simulink subsystem "RX"  (R2022b)
settings: Solver=VariableStepAuto  StartTime=0.0  StopTime=10.0  RelTol=1e-3
libraries: msbPllFoundation x2
settings Model: Creator=Ali-Laptop  LastModifiedBy=Ali-Laptop

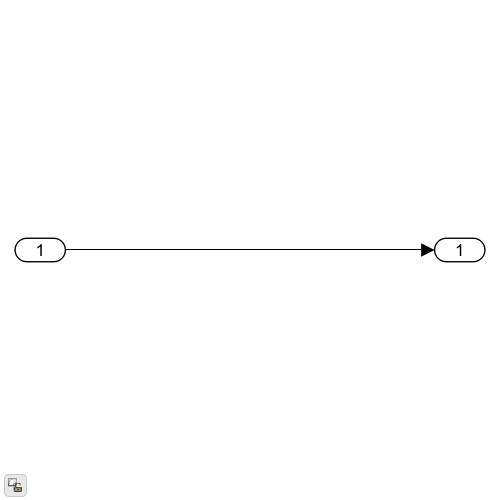
[thumbnail: Simulink's stored preview of the top-level diagram]
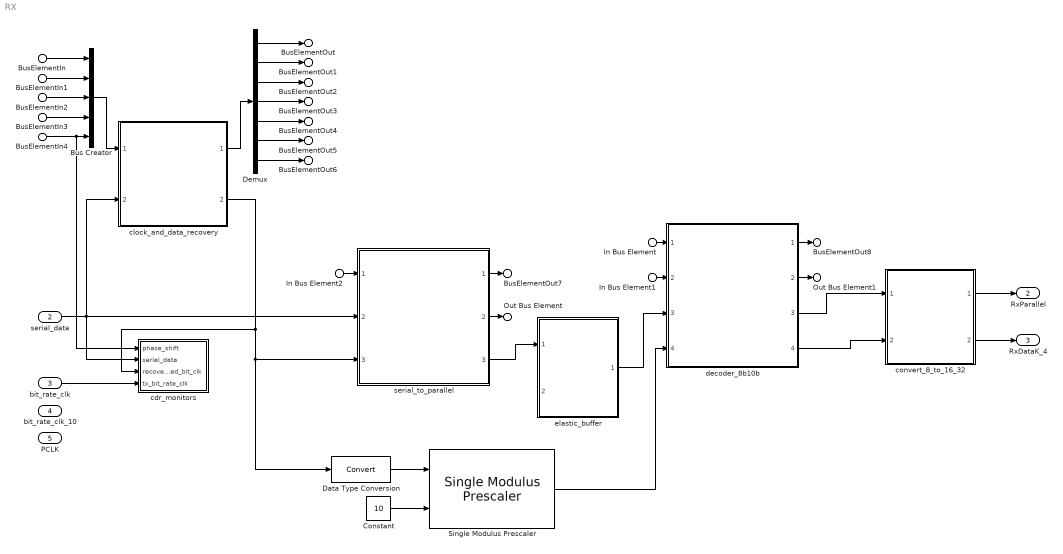
== system RX ==
  In Bus Element : Inport  PortName=digital_out  Element=RxDataK_out
  In Bus Element1 : Inport  PortName=digital_out  Element=RxParallel_8_out
  In Bus Element2 : Inport  PortName=digital_out  Element=RxParallel_10_out
  BusElementIn : Inport  PortName=digital_out  Element=Dn_out
  BusElementIn1 : Inport  PortName=digital_out  Element=Dn_1_out
  BusElementIn2 : Inport  PortName=digital_out  Element=Pn_out
  BusElementIn3 : Inport  PortName=digital_out  Element=decision_out
  BusElementIn4 : Inport  PortName=digital_out  Element=phase_shift
  serial_data : Inport  Port=2
  bit_rate_clk : Inport  Port=3
  bit_rate_clk_10 : Inport  Port=4
  PCLK : Inport  Port=5
  Bus Creator : BusCreator  Inputs=5
  Constant : Constant  Value=10
  Data Type Conversion : DataTypeConversion  SaturateOnIntegerOverflow=off  RndMeth=Floor
  Demux : Demux  Outputs=7
  Single Modulus Prescaler : msbPllFoundation/Single Modulus Prescaler  ExtraBuffer=off  NBuffer=1
  cdr_monitors : Subsystem
  clock_and_data_recovery : Subsystem  ReferencedSubsystem=clock_and_data_recovery
  convert_8_to_16_32 : Subsystem  ReferencedSubsystem=convert_8_to_16_32
  decoder_8b10b : Subsystem  ReferencedSubsystem=decoder_8b10b
  elastic_buffer : Subsystem  ReferencedSubsystem=elastic_buffer
  serial_to_parallel : Subsystem  ReferencedSubsystem=serial_to_parallel
  BusElementOut7 : Outport  PortName=digital_in  Element=RxBitCLK
  BusElementOut8 : Outport  PortName=digital_in  Element=RxBitCLK_10
  Out Bus Element : Outport  PortName=digital_in  Element=Serial_in
  Out Bus Element1 : Outport  PortName=digital_in  Element=RxParallel_10_in
  BusElementOut : Outport  PortName=digital_in  Element=data_clock
  BusElementOut1 : Outport  PortName=digital_in  Element=phase_clock
  BusElementOut2 : Outport  PortName=digital_in  Element=Dn_in
  BusElementOut3 : Outport  PortName=digital_in  Element=Dn_1_in
  BusElementOut4 : Outport  PortName=digital_in  Element=Pn_in
  BusElementOut5 : Outport  PortName=digital_in  Element=decision_in
  BusElementOut6 : Outport  PortName=digital_in  Element=recovered_clock
  RxParallel : Outport  Port=2
  RxDataK_4 : Outport  Port=3
  wires:
  elastic_buffer/1 -> decoder_8b10b/3
  convert_8_to_16_32/1 -> RxParallel/1
  clock_and_data_recovery/2 -> cdr_monitors/3(recovered_bit_clk), serial_to_parallel/3, Data Type Conversion/1
  serial_data/1 -> serial_to_parallel/2, cdr_monitors/2(serial_data), clock_and_data_recovery/2
  serial_to_parallel/2 -> Out Bus Element/1
  In Bus Element2/1 -> serial_to_parallel/1
  decoder_8b10b/2 -> Out Bus Element1/1
  decoder_8b10b/3 -> convert_8_to_16_32/1
  decoder_8b10b/4 -> convert_8_to_16_32/2
  In Bus Element/1 -> decoder_8b10b/1
  In Bus Element1/1 -> decoder_8b10b/2
  convert_8_to_16_32/2 -> RxDataK_4/1
  serial_to_parallel/3 -> elastic_buffer/1
  BusElementIn/1 -> Bus Creator/1
  BusElementIn1/1 -> Bus Creator/2
  BusElementIn2/1 -> Bus Creator/3
  BusElementIn3/1 -> Bus Creator/4
  BusElementIn4/1 -> Bus Creator/5, cdr_monitors/1(phase_shift)
  Bus Creator/1 -> clock_and_data_recovery/1
  Demux/1 -> BusElementOut/1
  Demux/2 -> BusElementOut1/1
  Demux/3 -> BusElementOut2/1
  Demux/4 -> BusElementOut3/1
  Demux/5 -> BusElementOut4/1
  Demux/6 -> BusElementOut5/1
  serial_to_parallel/1 -> BusElementOut7/1
  clock_and_data_recovery/1 -> Demux/1
  Demux/7 -> BusElementOut6/1
  decoder_8b10b/1 -> BusElementOut8/1
  Single Modulus Prescaler/1 -> decoder_8b10b/4
  Constant/1 -> Single Modulus Prescaler/2
  Data Type Conversion/1 -> Single Modulus Prescaler/1
  bit_rate_clk/1 -> cdr_monitors/4(tx_bit_rate_clk)

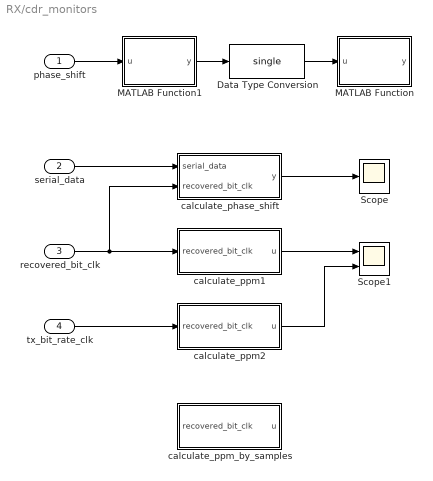
== system RX/cdr_monitors ==
  phase_shift : Inport
  serial_data : Inport  Port=2
  recovered_bit_clk : Inport  Port=3
  tx_bit_rate_clk : Inport  Port=4
  Data Type Conversion : DataTypeConversion  OutDataTypeStr=single  SaturateOnIntegerOverflow=off  RndMeth=Floor
  MATLAB Function : MATLAB Function  TreatAsAtomicUnit=on
  MATLAB Function1 : MATLAB Function  TreatAsAtomicUnit=on
  Scope : Scope
  Scope1 : Scope  NumInputPorts=2
  calculate_phase_shift : Subsystem
  calculate_ppm1 : Subsystem
  calculate_ppm2 : Subsystem
  calculate_ppm_by_samples : Subsystem
  wires:
  calculate_ppm2/1(u) -> Scope1/2
  tx_bit_rate_clk/1 -> calculate_ppm2/1(recovered_bit_clk)
  calculate_ppm1/1(u) -> Scope1/1
  Data Type Conversion/1 -> MATLAB Function/1(u)
  phase_shift/1 -> MATLAB Function1/1(u)
  MATLAB Function1/1(y) -> Data Type Conversion/1
  calculate_phase_shift/1(y) -> Scope/1
  recovered_bit_clk/1 -> calculate_ppm1/1(recovered_bit_clk), calculate_phase_shift/2(recovered_bit_clk)
  serial_data/1 -> calculate_phase_shift/1(serial_data)

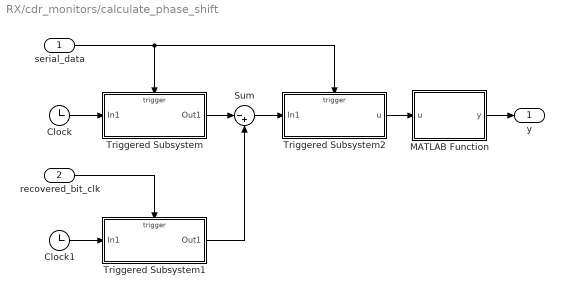
== system RX/cdr_monitors/calculate_phase_shift ==
  serial_data : Inport
  recovered_bit_clk : Inport  Port=2
  Clock : Clock
  Clock1 : Clock
  MATLAB Function : MATLAB Function  TreatAsAtomicUnit=on
  Sum : Sum  Inputs=|-+
  Triggered Subsystem : Subsystem  TreatAsAtomicUnit=on
  Triggered Subsystem1 : Subsystem  TreatAsAtomicUnit=on
  Triggered Subsystem2 : Subsystem  TreatAsAtomicUnit=on
  y : Outport
  wires:
  Triggered Subsystem2/1(u) -> MATLAB Function/1(u)
  MATLAB Function/1(y) -> y/1
  Sum/1 -> Triggered Subsystem2/1(In1)
  Triggered Subsystem1/1(Out1) -> Sum/2
  Triggered Subsystem/1(Out1) -> Sum/1
  serial_data/1 -> Triggered Subsystem/Trigger, Triggered Subsystem2/Trigger
  recovered_bit_clk/1 -> Triggered Subsystem1/Trigger
  Clock1/1 -> Triggered Subsystem1/1(In1)
  Clock/1 -> Triggered Subsystem/1(In1)

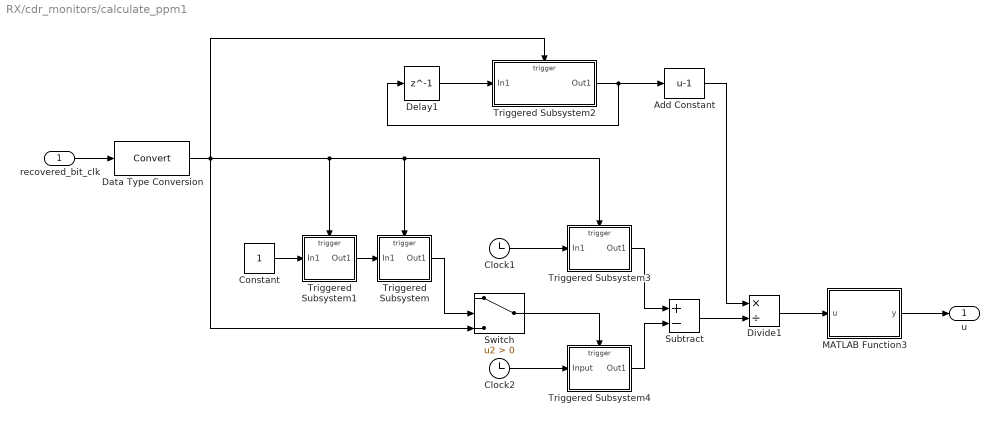
== system RX/cdr_monitors/calculate_ppm1 ==
  recovered_bit_clk : Inport
  Add Constant : Bias  Bias=-1  SaturateOnIntegerOverflow=off
  Clock1 : Clock
  Clock2 : Clock
  Constant : Constant
  Data Type Conversion : DataTypeConversion  SaturateOnIntegerOverflow=off  RndMeth=Floor
  Delay1 : Delay  DelayLength=1
  Divide1 : Product  Inputs=*/
  MATLAB Function3 : MATLAB Function  TreatAsAtomicUnit=on
  Subtract : Sum  Inputs=+-
  Switch : Switch  Criteria=u2 > Threshold  SaturateOnIntegerOverflow=off  InputSameDT=off
  Triggered Subsystem : Subsystem  TreatAsAtomicUnit=on
  Triggered Subsystem1 : Subsystem  TreatAsAtomicUnit=on
  Triggered Subsystem2 : Subsystem  TreatAsAtomicUnit=on
  Triggered Subsystem3 : Subsystem  TreatAsAtomicUnit=on
  Triggered Subsystem4 : Subsystem  TreatAsAtomicUnit=on
  u : Outport
  wires:
  Constant/1 -> Triggered Subsystem1/1(In1)
  MATLAB Function3/1(y) -> u/1
  Triggered Subsystem/1(Out1) -> Switch/2
  Triggered Subsystem1/1(Out1) -> Triggered Subsystem/1(In1)
  Divide1/1 -> MATLAB Function3/1(u)
  Data Type Conversion/1 -> Triggered Subsystem2/Trigger, Triggered Subsystem/Trigger, Triggered Subsystem3/Trigger, Triggered Subsystem1/Trigger, Switch/3
  Delay1/1 -> Triggered Subsystem2/1(In1)
  Triggered Subsystem4/1(Out1) -> Subtract/2
  Clock2/1 -> Triggered Subsystem4/1(Input)
  Switch/1 -> Triggered Subsystem4/Trigger
  Add Constant/1 -> Divide1/1
  recovered_bit_clk/1 -> Data Type Conversion/1
  Clock1/1 -> Triggered Subsystem3/1(In1)
  Triggered Subsystem3/1(Out1) -> Subtract/1
  Triggered Subsystem2/1(Out1) -> Add Constant/1, Delay1/1
  Subtract/1 -> Divide1/2

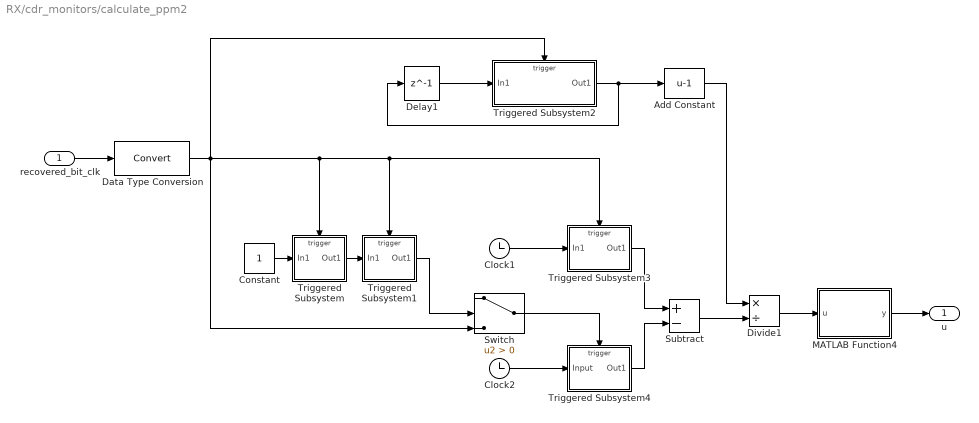
== system RX/cdr_monitors/calculate_ppm2 ==
  recovered_bit_clk : Inport
  Add Constant : Bias  Bias=-1  SaturateOnIntegerOverflow=off
  Clock1 : Clock
  Clock2 : Clock
  Constant : Constant
  Data Type Conversion : DataTypeConversion  SaturateOnIntegerOverflow=off  RndMeth=Floor
  Delay1 : Delay  DelayLength=1
  Divide1 : Product  Inputs=*/
  MATLAB Function4 : MATLAB Function  TreatAsAtomicUnit=on
  Subtract : Sum  Inputs=+-
  Switch : Switch  Criteria=u2 > Threshold  SaturateOnIntegerOverflow=off  InputSameDT=off
  Triggered Subsystem : Subsystem  TreatAsAtomicUnit=on
  Triggered Subsystem1 : Subsystem  TreatAsAtomicUnit=on
  Triggered Subsystem2 : Subsystem  TreatAsAtomicUnit=on
  Triggered Subsystem3 : Subsystem  TreatAsAtomicUnit=on
  Triggered Subsystem4 : Subsystem  TreatAsAtomicUnit=on
  u : Outport
  wires:
  MATLAB Function4/1(y) -> u/1
  Triggered Subsystem/1(Out1) -> Triggered Subsystem1/1(In1)
  Triggered Subsystem1/1(Out1) -> Switch/2
  Constant/1 -> Triggered Subsystem/1(In1)
  Divide1/1 -> MATLAB Function4/1(u)
  Data Type Conversion/1 -> Triggered Subsystem2/Trigger, Triggered Subsystem/Trigger, Triggered Subsystem3/Trigger, Triggered Subsystem1/Trigger, Switch/3
  Delay1/1 -> Triggered Subsystem2/1(In1)
  Triggered Subsystem4/1(Out1) -> Subtract/2
  Clock2/1 -> Triggered Subsystem4/1(Input)
  Switch/1 -> Triggered Subsystem4/Trigger
  Add Constant/1 -> Divide1/1
  recovered_bit_clk/1 -> Data Type Conversion/1
  Clock1/1 -> Triggered Subsystem3/1(In1)
  Triggered Subsystem3/1(Out1) -> Subtract/1
  Triggered Subsystem2/1(Out1) -> Add Constant/1, Delay1/1
  Subtract/1 -> Divide1/2

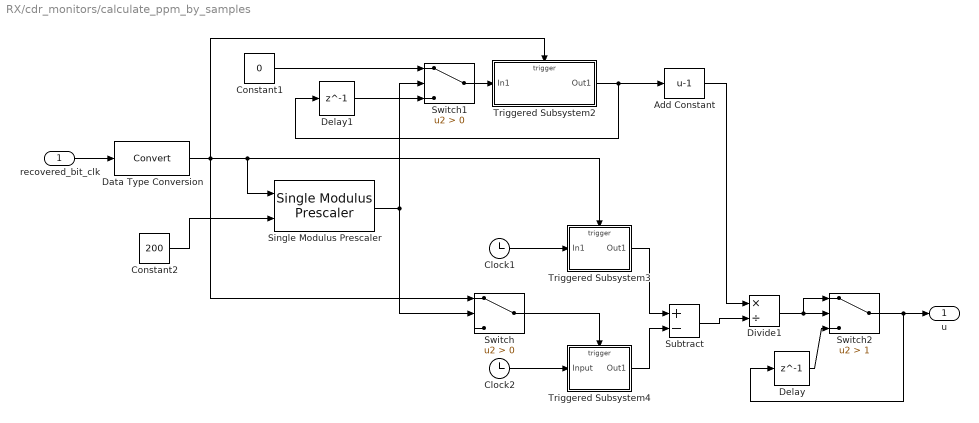
== system RX/cdr_monitors/calculate_ppm_by_samples ==
  recovered_bit_clk : Inport
  Add Constant : Bias  Bias=-1  SaturateOnIntegerOverflow=off
  Clock1 : Clock
  Clock2 : Clock
  Constant1 : Constant  Value=0
  Constant2 : Constant  Value=200
  Data Type Conversion : DataTypeConversion  SaturateOnIntegerOverflow=off  RndMeth=Floor
  Delay : Delay  DelayLength=1
  Delay1 : Delay  DelayLength=1
  Divide1 : Product  Inputs=*/
  Single Modulus Prescaler : msbPllFoundation/Single Modulus Prescaler  ExtraBuffer=off  NBuffer=1
  Subtract : Sum  Inputs=+-
  Switch : Switch  Criteria=u2 > Threshold  SaturateOnIntegerOverflow=off  InputSameDT=off
  Switch1 : Switch  Criteria=u2 > Threshold  SaturateOnIntegerOverflow=off  InputSameDT=off
  Switch2 : Switch  Criteria=u2 > Threshold  Threshold=1  SaturateOnIntegerOverflow=off  InputSameDT=off
  Triggered Subsystem2 : Subsystem  TreatAsAtomicUnit=on
  Triggered Subsystem3 : Subsystem  TreatAsAtomicUnit=on
  Triggered Subsystem4 : Subsystem  TreatAsAtomicUnit=on
  u : Outport
  wires:
  Switch2/1 -> Delay/1, u/1
  Delay/1 -> Switch2/3
  Divide1/1 -> Switch2/2, Switch2/1
  Single Modulus Prescaler/1 -> Switch1/2, Switch/2
  Data Type Conversion/1 -> Triggered Subsystem3/Trigger, Single Modulus Prescaler/1, Triggered Subsystem2/Trigger, Switch/1
  Constant2/1 -> Single Modulus Prescaler/2
  Constant1/1 -> Switch1/1
  Delay1/1 -> Switch1/3
  Switch1/1 -> Triggered Subsystem2/1(In1)
  Triggered Subsystem4/1(Out1) -> Subtract/2
  Clock2/1 -> Triggered Subsystem4/1(Input)
  Switch/1 -> Triggered Subsystem4/Trigger
  Add Constant/1 -> Divide1/1
  recovered_bit_clk/1 -> Data Type Conversion/1
  Clock1/1 -> Triggered Subsystem3/1(In1)
  Triggered Subsystem3/1(Out1) -> Subtract/1
  Triggered Subsystem2/1(Out1) -> Add Constant/1, Delay1/1
  Subtract/1 -> Divide1/2

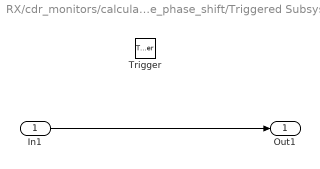
== system RX/cdr_monitors/calculate_phase_shift/Triggered Subsystem ==
  In1 : Inport
  Trigger : TriggerPort  TriggerType=either  VariantControl=(inherit)
  Out1 : Outport
  wires:
  In1/1 -> Out1/1

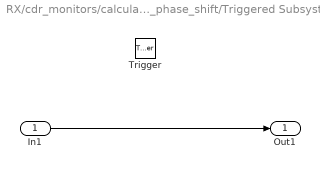
== system RX/cdr_monitors/calculate_phase_shift/Triggered Subsystem1 ==
  In1 : Inport
  Trigger : TriggerPort  TriggerType=falling  VariantControl=(inherit)
  Out1 : Outport
  wires:
  In1/1 -> Out1/1

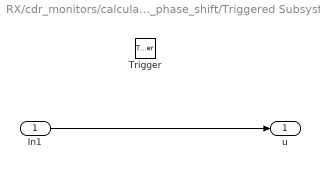
== system RX/cdr_monitors/calculate_phase_shift/Triggered Subsystem2 ==
  In1 : Inport
  Trigger : TriggerPort  VariantControl=(inherit)
  u : Outport
  wires:
  In1/1 -> u/1

== system RX/cdr_monitors/calculate_ppm1/Triggered Subsystem ==
  In1 : Inport
  Trigger : TriggerPort  TriggerType=falling  VariantControl=(inherit)
  Out1 : Outport
  wires:
  In1/1 -> Out1/1

== system RX/cdr_monitors/calculate_ppm1/Triggered Subsystem1 ==
  In1 : Inport
  Trigger : TriggerPort  VariantControl=(inherit)
  Out1 : Outport
  wires:
  In1/1 -> Out1/1

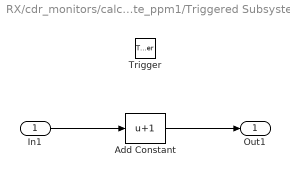
== system RX/cdr_monitors/calculate_ppm1/Triggered Subsystem2 ==
  In1 : Inport
  Trigger : TriggerPort  VariantControl=(inherit)
  Add Constant : Bias  Bias=1  SaturateOnIntegerOverflow=off
  Out1 : Outport
  wires:
  Add Constant/1 -> Out1/1
  In1/1 -> Add Constant/1

== system RX/cdr_monitors/calculate_ppm1/Triggered Subsystem3 ==
  In1 : Inport
  Trigger : TriggerPort  VariantControl=(inherit)
  Out1 : Outport
  wires:
  In1/1 -> Out1/1

== system RX/cdr_monitors/calculate_ppm1/Triggered Subsystem4 ==
  Input : Inport
  Trigger : TriggerPort  VariantControl=(inherit)
  Out1 : Outport
  wires:
  Input/1 -> Out1/1

== system RX/cdr_monitors/calculate_ppm2/Triggered Subsystem ==
  In1 : Inport
  Trigger : TriggerPort  VariantControl=(inherit)
  Out1 : Outport
  wires:
  In1/1 -> Out1/1

== system RX/cdr_monitors/calculate_ppm2/Triggered Subsystem1 ==
  In1 : Inport
  Trigger : TriggerPort  TriggerType=falling  VariantControl=(inherit)
  Out1 : Outport
  wires:
  In1/1 -> Out1/1

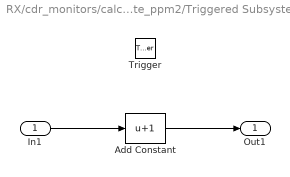
== system RX/cdr_monitors/calculate_ppm2/Triggered Subsystem2 ==
  In1 : Inport
  Trigger : TriggerPort  VariantControl=(inherit)
  Add Constant : Bias  Bias=1  SaturateOnIntegerOverflow=off
  Out1 : Outport
  wires:
  Add Constant/1 -> Out1/1
  In1/1 -> Add Constant/1

== system RX/cdr_monitors/calculate_ppm2/Triggered Subsystem3 ==
  In1 : Inport
  Trigger : TriggerPort  VariantControl=(inherit)
  Out1 : Outport
  wires:
  In1/1 -> Out1/1

== system RX/cdr_monitors/calculate_ppm2/Triggered Subsystem4 ==
  Input : Inport
  Trigger : TriggerPort  VariantControl=(inherit)
  Out1 : Outport
  wires:
  Input/1 -> Out1/1

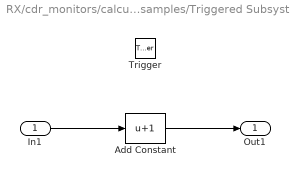
== system RX/cdr_monitors/calculate_ppm_by_samples/Triggered Subsystem2 ==
  In1 : Inport
  Trigger : TriggerPort  VariantControl=(inherit)
  Add Constant : Bias  Bias=1  SaturateOnIntegerOverflow=off
  Out1 : Outport
  wires:
  Add Constant/1 -> Out1/1
  In1/1 -> Add Constant/1

== system RX/cdr_monitors/calculate_ppm_by_samples/Triggered Subsystem3 ==
  In1 : Inport
  Trigger : TriggerPort  VariantControl=(inherit)
  Out1 : Outport
  wires:
  In1/1 -> Out1/1

== system RX/cdr_monitors/calculate_ppm_by_samples/Triggered Subsystem4 ==
  Input : Inport
  Trigger : TriggerPort  VariantControl=(inherit)
  Out1 : Outport
  wires:
  Input/1 -> Out1/1

== matlab function RX/cdr_monitors/MATLAB Function1 ==
  data: u input; y output
function y = fcn(u)

isNegative = int32(bitget(u,9));
y = int32(bitset(u,9,0)) + (-2^8)*isNegative;

== matlab function RX/cdr_monitors/MATLAB Function ==
  data: u input; y output
function y = fcn(u)

y = u*360/512;

== matlab function RX/cdr_monitors/calculate_ppm1/MATLAB Function3 ==
  data: u input; y output
function y = fcn(u)

y = (u-5e9)*1e6/5e9;

== matlab function RX/cdr_monitors/calculate_ppm2/MATLAB Function4 ==
  data: u input; y output
function y = fcn(u)

y = (u-5e9)*1e6/5e9;

== matlab function RX/cdr_monitors/calculate_phase_shift/MATLAB Function ==
  data: u input; y output
function y = fcn(u)

UI = 2e-10;

phase = (360*u)/UI;

if phase >= -180
    y = phase;
else
    y = phase + 360;
end
